simulink model "ev_pv_smoothing"  (Simulink 8.1)
settings: Solver=ode3  StartTime=0  StopTime=86400  FixedStep=15  RelTol=1e-3
undefined symbols (not defined in the file or in its folder): D1, Delta, SRRL, Ts, Weather
libraries: CampusEnergyModeling x22, powerlib x9, simulink x4, powerlib_meascontrol x4
settings Model: Creator=sfrank1  LastModifiedBy=sfrank1
settings DataIOCC: SignalLoggingSaveFormat=Dataset
settings OptimizationCC: ExpressionDepthLimit=128
settings DebuggingCC: FcnCallInpInsideContextMsg=EnableAllAsError
settings GRTTargetCC: CombineOutputUpdateFcns=on  GRTInterface=off

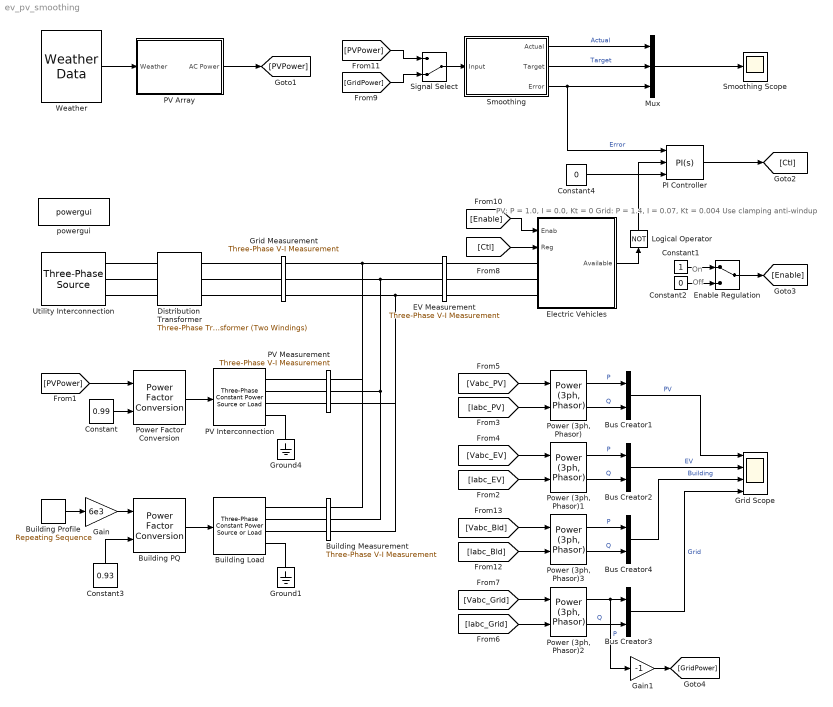
== system ev_pv_smoothing ==
  note: PV: P = 1.0, I = 0.0, Kt = 0
      | Grid: P = 1.4, I = 0.07, Kt = 0.004
      | Use clamping anti-windup
  note: Off
  note: On
  Building Measurement : powerlib/Measurements/Three-Phase V-I Measurement  VoltageMeasurement=phase-to-ground  SetLabelV=on  LabelV=Vabc_Bld  Vpu=off  VpuLL=off  CurrentMeasurement=yes  SetLabelI=on  LabelI=Iabc_Bld  Ipu=off  Pbase=100e3  Vbase=208e3  OutputType=Complex  PhasorSimulation=on  PSBequivalent=0
  Building Profile : simulink/Sources/Repeating Sequence  rep_seq_t=[0 1 2 3 4 5 6 7 8 9 10 11 12 13 14 15 16 17 18 19 20 21 22 23 24]*3600  rep_seq_y=[0.53 0.53 0.54 0.54 0.56 0.77 0.95 1.53 1.79 1.80 1.83 1.83 1.88 1.91 1.91 1.92 1.63 1.28 1.20 1.13 1.08 0.71 0.52 0.52 0.53]
  Building Load : CampusEnergyModeling/Electrical/Three-Phase Constant Power Source or Load  Conven=load  PNom=5e3  QNom=2e3  VNom=208  fNom=60  VLow=0.7
  Building PQ : CampusEnergyModeling/Electrical/Power Factor Conversion  pfType=Lagging
  Bus Creator{1..4} (4 alike) : BusCreator  Inputs=2
  Constant : Constant  Value=0.99
  Constant1 : Constant
  Constant2 : Constant  Value=0
  Constant3 : Constant  Value=0.93
  Constant4 : Constant  Value=0
  Distribution Transformer : powerlib/Elements/Three-Phase Transformer (Two Windings)  Winding1Connection=Delta (D1)  UNITS=pu  NominalPower=[10e3 , 60]  Winding1=[13.2e3 , 0.02/2 , 0.05/(120*pi)/2]  Winding2Connection=Yg  Winding2=[208, 0.02/2 , 0.05/(120*pi)/2]  SetSaturation=off  Rm=500  Lm=200  Saturation=[ 0,0 ; 0.0024,1.2 ; 1.0,1.52 ]  Hysteresis=off  DataFile='hysteresis'  SetInitialFlux=off  InitialFluxes=[ 0.8 , -0.8 , 0.7 ]  Measurements=None  MoreParameters=off  BreakLoop=off  DataType=off  TransfoNumber=1
  EV Measurement : powerlib/Measurements/Three-Phase V-I Measurement  VoltageMeasurement=phase-to-ground  SetLabelV=on  LabelV=Vabc_EV  Vpu=off  VpuLL=off  CurrentMeasurement=yes  SetLabelI=on  LabelI=Iabc_EV  Ipu=off  Pbase=100e3  Vbase=208e3  OutputType=Complex  PhasorSimulation=on  PSBequivalent=0
  Electric Vehicles : Subsystem
  Enable Regulation : ManualSwitch
  Gain : Gain  Gain=6e3
  Gain1 : Gain  Gain=-1
  Grid Measurement : powerlib/Measurements/Three-Phase V-I Measurement  VoltageMeasurement=phase-to-ground  SetLabelV=on  LabelV=Vabc_Grid  Vpu=off  VpuLL=off  CurrentMeasurement=yes  SetLabelI=on  LabelI=Iabc_Grid  Ipu=off  Pbase=100e3  Vbase=208e3  OutputType=Complex  PhasorSimulation=on  PSBequivalent=0
  Grid Scope : Scope  NumInputPorts=4
      settings: ShowLegends=on  TimeRange=86400  YMin=-5000~-5000~-5000~-5000  YMax=25000~25000~25000~25000
  Ground1 : powerlib/Elements/Ground  LConnTagsString=a
  Ground4 : powerlib/Elements/Ground  LConnTagsString=a
  Logical Operator : Logic  Operator=NOT  IconShape=distinctive  AllPortsSameDT=off  OutDataTypeStr=boolean
  Mux : Mux  Inputs=3
  PI Controller : simulink/Continuous/PID Controller  Controller=PI  TimeDomain=Continuous-time  SampleTime=1  IntegratorMethod=Forward Euler  FilterMethod=Forward Euler  Form=Parallel  P=1.4  I=0.07  D=0  N=100  InitialConditionSource=internal  InitialConditionForIntegrator=0  InitialConditionForFilter=0  ExternalReset=level  ZeroCross=off  LimitOutput=on  UpperSaturationLimit=12e3  LowerSaturationLimit=-12e3  LinearizeAsGain=on  AntiWindupMode=clamping  Kb=1  TrackingMode=on  Kt=0.004  PParamMin=[]  PParamMax=[]  IParamMin=[]  IParamMax=[]  DParamMin=[]  DParamMax=[]  NParamMin=[]  NParamMax=[]  KbParamMin=[]  KbParamMax=[]  KtParamMin=[]  KtParamMax=[]  POutMin=[]  POutMax=[]  IOutMin=[]  IOutMax=[]  DOutMin=[]  DOutMax=[]  NOutMin=[]  NOutMax=[]  KbOutMin=[]  KbOutMax=[]  KtOutMin=[]  KtOutMax=[]  IntegratorOutMin=[]  IntegratorOutMax=[]  FilterOutMin=[]  FilterOutMax=[]  SumOutMin=[]  SumOutMax=[]  SumI1OutMin=[]  SumI1OutMax=[]  SumI2OutMin=[]  SumI2OutMax=[]  SumI3OutMin=[]  SumI3OutMax=[]  SumDOutMin=[]  SumDOutMax=[]  SaturationOutMin=[]  SaturationOutMax=[]  IntegratorContinuousStateAttributes=''  IntegratorStateMustResolveToSignalObject=off  IntegratorRTWStateStorageClass=Auto  FilterContinuousStateAttributes=''  FilterStateMustResolveToSignalObject=off  FilterRTWStateStorageClass=Auto
  PV Interconnection : CampusEnergyModeling/Electrical/Three-Phase Constant Power Source or Load  Conven=source  PNom=20e3  QNom=0  VNom=208  fNom=60  VLow=0.7
  PV Array : Subsystem
  PV Measurement : powerlib/Measurements/Three-Phase V-I Measurement  VoltageMeasurement=phase-to-ground  SetLabelV=on  LabelV=Vabc_PV  Vpu=off  VpuLL=off  CurrentMeasurement=yes  SetLabelI=on  LabelI=Iabc_PV  Ipu=off  Pbase=100e3  Vbase=208e3  OutputType=Complex  PhasorSimulation=on  PSBequivalent=0
  Power (3ph, Phasor){,1..3} (4 alike) : powerlib_meascontrol/Measurements/Power (3ph, Phasor)
  Power Factor Conversion : CampusEnergyModeling/Electrical/Power Factor Conversion  pfType=Lagging
  Signal Select : ManualSwitch  CurrentSetting=0
  Smoothing : Subsystem
  Smoothing Scope : Scope
      settings: ShowLegends=on  TimeRange=86400  YMin=-20000  YMax=20000
  Utility Interconnection : powerlib/Electrical Sources/Three-Phase Source  Voltage=13.2e3  PhaseAngle=0  Frequency=60  InternalConnection=Yg  SpecifyImpedance=on  Resistance=0.8929  Inductance=16.58e-3  ShortCircuitLevel=1e6  BaseVoltage=13.2e3  XRratio=8  BusType=swing  Pref=0  Qref=0  Qmin=-inf  Qmax=inf
  Weather : CampusEnergyModeling/Weather/Weather Data  fname=Weather-SRRL.mat  initbus=on
  powergui : powerlib/powergui  Priority=2  SimulationMode=Phasor  SolverType=Tustin  SampleTime=Ts  frequency=60  SPID=off  DisableSnubberDevices=off  DisableRonSwitches=off  DisableVfSwitches=off  SwTol=0  Interpol=off  DisplayEquations=off  frequencyindice=60  Pbase=100e6  ErrMax=1e-4  Iterations=50  UnitsV=kV  UnitsW=kW  FunctionMessages=off  echomessages=off  HookPort=off  EnableUseOfTLC=off  x0status=blocks  RestoreLinks=warning  ResistiveCurrentMeasurement=off  Frange=[0:2:500]  Ylog=off  Xlog=on  ShowGrid=off  save=off  variable=ZData  structure=Sig1  ZoomFFT=on  StartTime=0.26  cycles=2  DisplayStyle=1  fundamental=60  FreqAxis=off  MaxFrequency=5000  frequencyindicesteady=1  RmsSteady=1  display=off  Ts=0  methode=off
  wires:
  Smoothing/3(Error) -> PI Controller/1, Mux/3  "Error"
  Mux/1 -> Smoothing Scope/1
  Smoothing/1(Actual) -> Mux/1  "Actual"
  Smoothing/2(Target) -> Mux/2  "Target"
  Constant/1 -> Power Factor Conversion/2
  Power Factor Conversion/1 -> PV Interconnection/1
  [Vabc_PV] -> "Power (3ph, Phasor)"/1
  [Iabc_PV] -> "Power (3ph, Phasor)"/2
  "Power (3ph, Phasor)"/2 -> Bus Creator1/2  "Q"
  "Power (3ph, Phasor)"/1 -> Bus Creator1/1  "P"
  Bus Creator1/1 -> Grid Scope/1  "PV"
  [Vabc_EV] -> "Power (3ph, Phasor)1"/1
  [Iabc_EV] -> "Power (3ph, Phasor)1"/2
  "Power (3ph, Phasor)1"/2 -> Bus Creator2/2  "Q"
  "Power (3ph, Phasor)1"/1 -> Bus Creator2/1  "P"
  [Vabc_Grid] -> "Power (3ph, Phasor)2"/1
  [Iabc_Grid] -> "Power (3ph, Phasor)2"/2
  "Power (3ph, Phasor)2"/2 -> Bus Creator3/2  "Q"
  "Power (3ph, Phasor)2"/1 -> Gain1/1, Bus Creator3/1  "P"
  Bus Creator3/1 -> Grid Scope/4  "Grid"
  Bus Creator2/1 -> Grid Scope/2  "EV"
  Constant1/1 -> Enable Regulation/1
  Constant2/1 -> Enable Regulation/2
  Weather/1 -> PV Array/1(Weather)
  [PVPower] -> Power Factor Conversion/1
  [Ctl] -> Electric Vehicles/2(Reg)
  Enable Regulation/1 -> [Enable]
  [Enable] -> Electric Vehicles/1(Enab)
  Building PQ/1 -> Building Load/1
  Building Profile/1 -> Gain/1
  [Vabc_Bld] -> "Power (3ph, Phasor)3"/1
  [Iabc_Bld] -> "Power (3ph, Phasor)3"/2
  "Power (3ph, Phasor)3"/2 -> Bus Creator4/2  "Q"
  "Power (3ph, Phasor)3"/1 -> Bus Creator4/1  "P"
  Bus Creator4/1 -> Grid Scope/3  "Building"
  Gain/1 -> Building PQ/1
  Constant3/1 -> Building PQ/2
  Electric Vehicles/1(Available) -> Logical Operator/1
  Signal Select/1 -> Smoothing/1(Input)
  [PVPower] -> Signal Select/1
  [GridPower] -> Signal Select/2
  Logical Operator/1 -> PI Controller/2
  PI Controller/1 -> [Ctl]
  Gain1/1 -> [GridPower]
  PV Array/1(AC Power) -> [PVPower]
  Constant4/1 -> PI Controller/3
  connections:
  Utility Interconnection/RConn1 -- Distribution Transformer/LConn1
  Distribution Transformer/LConn2 -- Utility Interconnection/RConn2
  Utility Interconnection/RConn3 -- Distribution Transformer/LConn3
  EV Measurement/LConn1 -- Building Measurement/LConn1 -- PV Measurement/RConn1 -- Grid Measurement/RConn1
  PV Measurement/RConn2 -- EV Measurement/LConn2 -- Grid Measurement/RConn2 -- Building Measurement/LConn2
  EV Measurement/LConn3 -- Building Measurement/LConn3 -- PV Measurement/RConn3 -- Grid Measurement/RConn3
  PV Interconnection/RConn4 -- Ground4/LConn1
  PV Measurement/LConn1 -- PV Interconnection/RConn1
  PV Measurement/LConn2 -- PV Interconnection/RConn2
  PV Measurement/LConn3 -- PV Interconnection/RConn3
  EV Measurement/RConn1 -- Electric Vehicles/LConn1
  EV Measurement/RConn2 -- Electric Vehicles/LConn2
  EV Measurement/RConn3 -- Electric Vehicles/LConn3
  Building Load/RConn4 -- Ground1/LConn1
  Distribution Transformer/RConn1 -- Grid Measurement/LConn1
  Distribution Transformer/RConn2 -- Grid Measurement/LConn2
  Distribution Transformer/RConn3 -- Grid Measurement/LConn3
  Building Load/RConn1 -- Building Measurement/RConn1
  Building Load/RConn2 -- Building Measurement/RConn2
  Building Load/RConn3 -- Building Measurement/RConn3

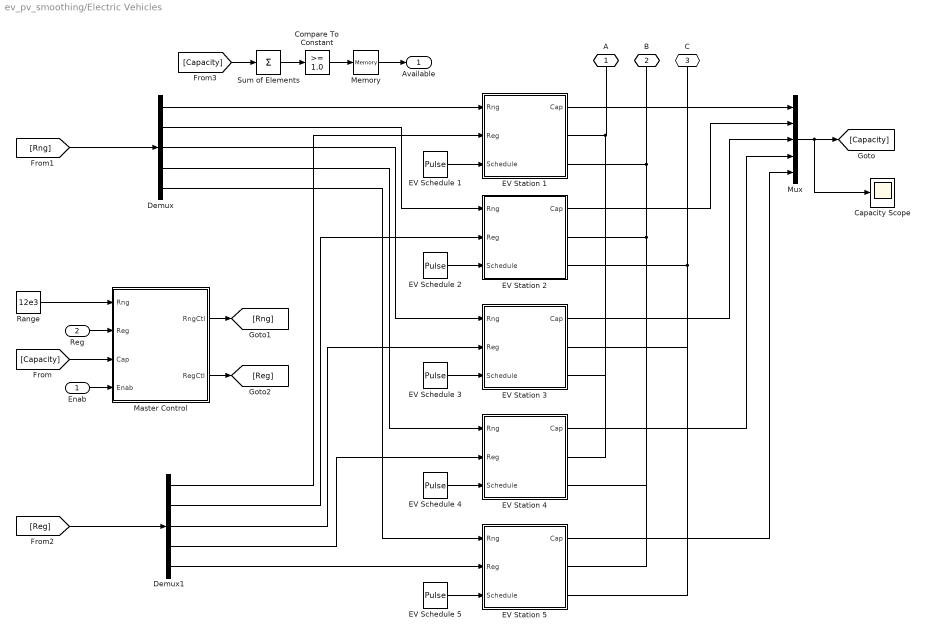
== system ev_pv_smoothing/Electric Vehicles ==
  Enab : Inport
  Reg : Inport  Port=2
  Capacity Scope : Scope
      settings: ShowLegends=on  TimeRange=86400  YMin=0  YMax=3000  SaveName=ScopeData3
  Compare To Constant : simulink/Logic and Bit Operations/Compare To Constant  relop=>=  const=1.0  OutDataTypeStr=boolean
  Demux : Demux  Outputs=5
  Demux1 : Demux  Outputs=5
  EV Schedule 1 : DiscretePulseGenerator  PulseType=Time based  Period=86400  PulseWidth=(9/24)*100  PhaseDelay=(6)*3600
  EV Schedule 2 : DiscretePulseGenerator  PulseType=Time based  Period=86400  PulseWidth=(9/24)*100  PhaseDelay=(6.5)*3600
  EV Schedule 3 : DiscretePulseGenerator  PulseType=Time based  Period=86400  PulseWidth=(9/24)*100  PhaseDelay=(7)*3600
  EV Schedule 4 : DiscretePulseGenerator  PulseType=Time based  Period=86400  PulseWidth=(9/24)*100  PhaseDelay=(7.5)*3600
  EV Schedule 5 : DiscretePulseGenerator  PulseType=Time based  Period=86400  PulseWidth=(9/24)*100  PhaseDelay=(8)*3600
  EV Station 1 : Subsystem
  EV Station 2 : Subsystem
  EV Station 3 : Subsystem
  EV Station 4 : Subsystem
  EV Station 5 : Subsystem
  Master Control : Subsystem
  Memory : Memory
  Mux : Mux  Inputs=5
  Range : Constant  Value=12e3
  Sum of Elements : Sum  Inputs=+
  A : PMIOPort  Port=1  Side=Left
  B : PMIOPort  Port=2  Side=Left
  C : PMIOPort  Port=3  Side=Left
  Available : Outport
  wires:
  EV Schedule 1/1 -> EV Station 1/3(Schedule)
  EV Schedule 2/1 -> EV Station 2/3(Schedule)
  EV Schedule 3/1 -> EV Station 3/3(Schedule)
  EV Schedule 4/1 -> EV Station 4/3(Schedule)
  EV Schedule 5/1 -> EV Station 5/3(Schedule)
  Range/1 -> Master Control/1(Rng)
  Reg/1 -> Master Control/2(Reg)
  Enab/1 -> Master Control/4(Enab)
  EV Station 1/1(Cap) -> Mux/1
  EV Station 2/1(Cap) -> Mux/2
  EV Station 3/1(Cap) -> Mux/3
  EV Station 4/1(Cap) -> Mux/4
  EV Station 5/1(Cap) -> Mux/5
  Mux/1 -> Capacity Scope/1, [Capacity]
  [Capacity] -> Master Control/3(Cap)
  Master Control/2(RegCtl) -> [Reg]
  Master Control/1(RngCtl) -> [Rng]
  [Rng] -> Demux/1
  [Reg] -> Demux1/1
  Demux/1 -> EV Station 1/1(Rng)
  Demux1/5 -> EV Station 5/2(Reg)
  Demux/2 -> EV Station 2/1(Rng)
  Demux/3 -> EV Station 3/1(Rng)
  Demux/4 -> EV Station 4/1(Rng)
  Demux/5 -> EV Station 5/1(Rng)
  Demux1/1 -> EV Station 1/2(Reg)
  Demux1/2 -> EV Station 2/2(Reg)
  Demux1/3 -> EV Station 3/2(Reg)
  Demux1/4 -> EV Station 4/2(Reg)
  Sum of Elements/1 -> Compare To Constant/1
  [Capacity] -> Sum of Elements/1
  Compare To Constant/1 -> Memory/1
  Memory/1 -> Available/1
  connections:
  EV Station 1/RConn2 -- EV Station 2/RConn1 -- EV Station 5/RConn1 -- EV Station 4/RConn2 -- B/RConn1
  EV Station 5/RConn2 -- EV Station 3/RConn1 -- EV Station 2/RConn2 -- C/RConn1
  EV Station 1/RConn1 -- EV Station 4/RConn1 -- EV Station 3/RConn2 -- A/RConn1

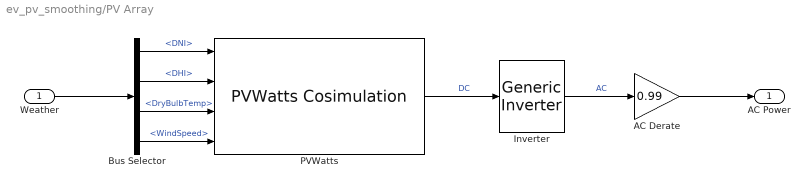
== system ev_pv_smoothing/PV Array ==
  Weather : Inport
  AC Derate : Gain  Gain=0.99
  Bus Selector : BusSelector  OutputSignals=DNI,DHI,DryBulbTemp,WindSpeed
  Inverter : CampusEnergyModeling/PV/Generic Inverter  max_power=20.0e3  standby=10.0  model_type=Fixed Efficiency  fixed_eff=0.96  alpha=100.0  beta=0.04  gamma=4.0e-07  lookup_pair=Input Power + Output Power  lookup_in=[0, 10, 25, 50, 75, 100]  lookup_out=[0, 9, 24, 49, 73, 97]  lookup_eff=[0.10, 0.80, 0.87, 0.93, 0.90, 0.88]
  PVWatts : CampusEnergyModeling/PV/PVWatts Cosimulation  lat=39.7  lon=-105.2  start_time=2012-05-17 00:00:00  tz=-7  time_step=15  system_size=20.0e3  derate=0.908  azimuth=180  tilt=10  use_lat_tilt=off  track_mode=Fixed  rotlim=45  use_cell_data=off  t_ref=25  t_noct=45  gamma=-0.5  i_ref=1000  poa_cutin=0  init_tcell=16.8  init_poa=0  alignment=Middle  output_dc=on  output_celltemp=off  output_poa=off
  AC Power : Outport
  wires:
  Bus Selector/1 -> PVWatts/1  "<DNI>"
  Bus Selector/2 -> PVWatts/2  "<DHI>"
  Bus Selector/3 -> PVWatts/3  "<DryBulbTemp>"
  Bus Selector/4 -> PVWatts/4  "<WindSpeed>"
  PVWatts/1 -> Inverter/1  "DC"
  Inverter/1 -> AC Derate/1  "AC"
  AC Derate/1 -> AC Power/1
  Weather/1 -> Bus Selector/1

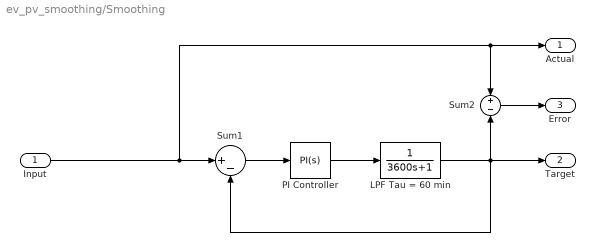
== system ev_pv_smoothing/Smoothing ==
  Input : Inport
  LPF Tau = 60 min : TransferFcn  Denominator=[3600 1]
  PI Controller : simulink/Continuous/PID Controller  Controller=PI  TimeDomain=Continuous-time  SampleTime=1  IntegratorMethod=Forward Euler  FilterMethod=Forward Euler  Form=Parallel  P=0.80  I=0.001  D=0  N=100  InitialConditionSource=internal  InitialConditionForIntegrator=0  InitialConditionForFilter=0  ExternalReset=none  LimitOutput=off  UpperSaturationLimit=20e3  LowerSaturationLimit=-20e3  LinearizeAsGain=on  AntiWindupMode=back-calculation  Kb=1  TrackingMode=off  Kt=1  PParamMin=[]  PParamMax=[]  IParamMin=[]  IParamMax=[]  DParamMin=[]  DParamMax=[]  NParamMin=[]  NParamMax=[]  KbParamMin=[]  KbParamMax=[]  KtParamMin=[]  KtParamMax=[]  POutMin=[]  POutMax=[]  IOutMin=[]  IOutMax=[]  DOutMin=[]  DOutMax=[]  NOutMin=[]  NOutMax=[]  KbOutMin=[]  KbOutMax=[]  KtOutMin=[]  KtOutMax=[]  IntegratorOutMin=[]  IntegratorOutMax=[]  FilterOutMin=[]  FilterOutMax=[]  SumOutMin=[]  SumOutMax=[]  SumI1OutMin=[]  SumI1OutMax=[]  SumI2OutMin=[]  SumI2OutMax=[]  SumI3OutMin=[]  SumI3OutMax=[]  SumDOutMin=[]  SumDOutMax=[]  SaturationOutMin=[]  SaturationOutMax=[]  IntegratorContinuousStateAttributes=''  IntegratorStateMustResolveToSignalObject=off  IntegratorRTWStateStorageClass=Auto  FilterContinuousStateAttributes=''  FilterStateMustResolveToSignalObject=off  FilterRTWStateStorageClass=Auto
  Sum1 : Sum  Inputs=|+-
  Sum2 : Sum  Inputs=+-
  Actual : Outport
  Target : Outport  Port=2
  Error : Outport  Port=3
  wires:
  Sum2/1 -> Error/1
  LPF Tau = 60 min/1 -> Sum1/2, Target/1, Sum2/2
  Input/1 -> Sum2/1, Actual/1, Sum1/1
  PI Controller/1 -> LPF Tau = 60 min/1
  Sum1/1 -> PI Controller/1

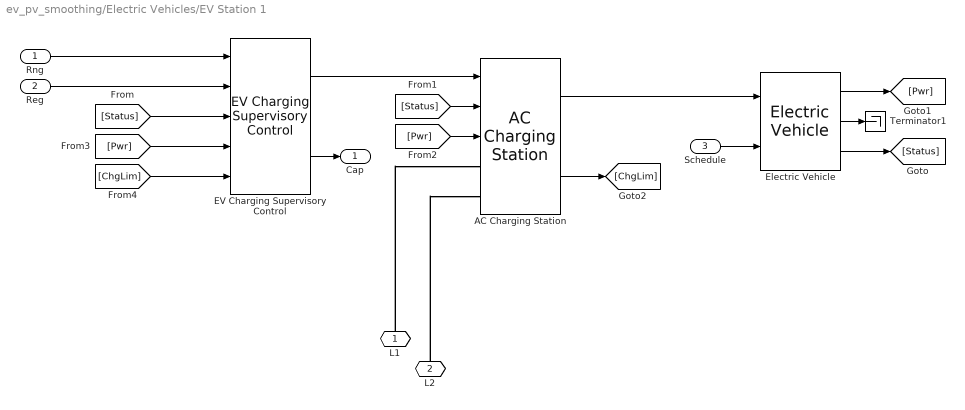
== system ev_pv_smoothing/Electric Vehicles/EV Station 1 ==
  Rng : Inport
  Reg : Inport  Port=2
  Schedule : Inport  Port=3
  AC Charging Station : CampusEnergyModeling/Electric Vehicles/AC Charging Station  prated=6600  vrated=240  pstandby=50  eff=0.99  pf=0.99  freq=60
  EV Charging Supervisory Control : CampusEnergyModeling/Electric Vehicles/EV Charging Supervisory Control  ctype=AC  ramp=100  regtype=Two-sided  ldsettings=on  sweepint=1650+300*rand(1)  sweepramp=10  thr=1.0
  Electric Vehicle : CampusEnergyModeling/Electric Vehicles/Electric Vehicle  ctype=AC  rating=6240  chargerEff=0.96  profile=off  profileSOC=[0.00 0.10 0.20 0.80 0.99 1.00]  profileRate=[0.10 0.20 1.00 1.00 0.01 0.00]  capacity=24000  initSOC=0.3  battEff=0.98
  Terminator1 : Terminator
  L1 : PMIOPort  Port=1  Side=Right
  L2 : PMIOPort  Port=2  Side=Right
  Cap : Outport
  wires:
  AC Charging Station/1 -> Electric Vehicle/1
  Schedule/1 -> Electric Vehicle/2
  Electric Vehicle/3 -> [Status]
  [Status] -> EV Charging Supervisory Control/3
  Electric Vehicle/1 -> [Pwr]
  EV Charging Supervisory Control/1 -> AC Charging Station/1
  [Status] -> AC Charging Station/2
  [Pwr] -> AC Charging Station/3
  Reg/1 -> EV Charging Supervisory Control/2
  Rng/1 -> EV Charging Supervisory Control/1
  EV Charging Supervisory Control/2 -> Cap/1
  Electric Vehicle/2 -> Terminator1/1
  [Pwr] -> EV Charging Supervisory Control/4
  [ChgLim] -> EV Charging Supervisory Control/5
  AC Charging Station/2 -> [ChgLim]
  connections:
  L1/RConn1 -- AC Charging Station/LConn1
  L2/RConn1 -- AC Charging Station/LConn2

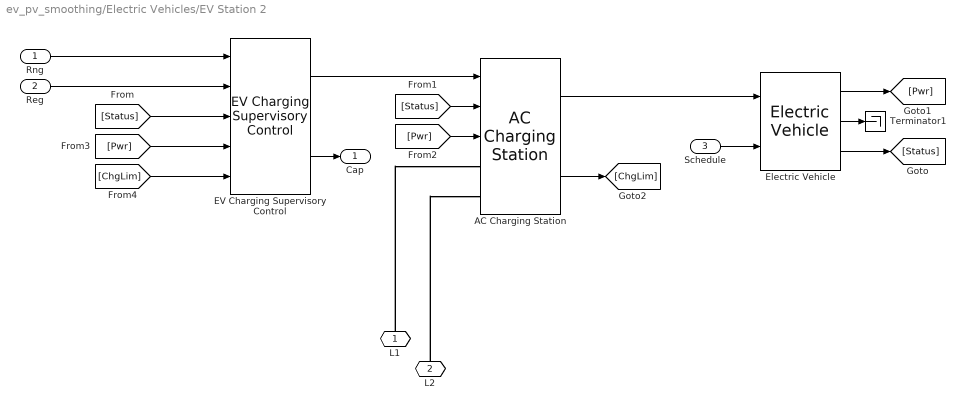
== system ev_pv_smoothing/Electric Vehicles/EV Station 2 ==
  Rng : Inport
  Reg : Inport  Port=2
  Schedule : Inport  Port=3
  AC Charging Station : CampusEnergyModeling/Electric Vehicles/AC Charging Station  prated=6600  vrated=240  pstandby=50  eff=0.99  pf=0.99  freq=60
  EV Charging Supervisory Control : CampusEnergyModeling/Electric Vehicles/EV Charging Supervisory Control  ctype=AC  ramp=100  regtype=Two-sided  ldsettings=on  sweepint=1650+300*rand(1)  sweepramp=10  thr=1.0
  Electric Vehicle : CampusEnergyModeling/Electric Vehicles/Electric Vehicle  ctype=AC  rating=6240  chargerEff=0.96  profile=off  profileSOC=[0.00 0.10 0.20 0.80 0.99 1.00]  profileRate=[0.10 0.20 1.00 1.00 0.01 0.00]  capacity=24000  initSOC=0.3  battEff=0.98
  Terminator1 : Terminator
  L1 : PMIOPort  Port=1  Side=Right
  L2 : PMIOPort  Port=2  Side=Right
  Cap : Outport
  wires:
  AC Charging Station/1 -> Electric Vehicle/1
  Schedule/1 -> Electric Vehicle/2
  Electric Vehicle/3 -> [Status]
  [Status] -> EV Charging Supervisory Control/3
  Electric Vehicle/1 -> [Pwr]
  EV Charging Supervisory Control/1 -> AC Charging Station/1
  [Status] -> AC Charging Station/2
  [Pwr] -> AC Charging Station/3
  Reg/1 -> EV Charging Supervisory Control/2
  Rng/1 -> EV Charging Supervisory Control/1
  EV Charging Supervisory Control/2 -> Cap/1
  Electric Vehicle/2 -> Terminator1/1
  [Pwr] -> EV Charging Supervisory Control/4
  [ChgLim] -> EV Charging Supervisory Control/5
  AC Charging Station/2 -> [ChgLim]
  connections:
  L1/RConn1 -- AC Charging Station/LConn1
  L2/RConn1 -- AC Charging Station/LConn2

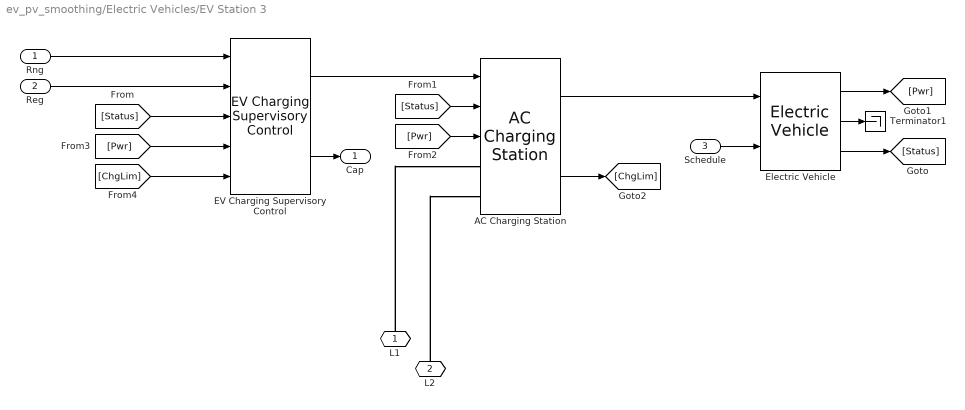
== system ev_pv_smoothing/Electric Vehicles/EV Station 3 ==
  Rng : Inport
  Reg : Inport  Port=2
  Schedule : Inport  Port=3
  AC Charging Station : CampusEnergyModeling/Electric Vehicles/AC Charging Station  prated=6600  vrated=240  pstandby=50  eff=0.99  pf=0.99  freq=60
  EV Charging Supervisory Control : CampusEnergyModeling/Electric Vehicles/EV Charging Supervisory Control  ctype=AC  ramp=100  regtype=Two-sided  ldsettings=on  sweepint=1650+300*rand(1)  sweepramp=10  thr=1.0
  Electric Vehicle : CampusEnergyModeling/Electric Vehicles/Electric Vehicle  ctype=AC  rating=6240  chargerEff=0.96  profile=off  profileSOC=[0.00 0.10 0.20 0.80 0.99 1.00]  profileRate=[0.10 0.20 1.00 1.00 0.01 0.00]  capacity=24000  initSOC=0.3  battEff=0.98
  Terminator1 : Terminator
  L1 : PMIOPort  Port=1  Side=Right
  L2 : PMIOPort  Port=2  Side=Right
  Cap : Outport
  wires:
  AC Charging Station/1 -> Electric Vehicle/1
  Schedule/1 -> Electric Vehicle/2
  Electric Vehicle/3 -> [Status]
  [Status] -> EV Charging Supervisory Control/3
  Electric Vehicle/1 -> [Pwr]
  EV Charging Supervisory Control/1 -> AC Charging Station/1
  [Status] -> AC Charging Station/2
  [Pwr] -> AC Charging Station/3
  Reg/1 -> EV Charging Supervisory Control/2
  Rng/1 -> EV Charging Supervisory Control/1
  EV Charging Supervisory Control/2 -> Cap/1
  Electric Vehicle/2 -> Terminator1/1
  [Pwr] -> EV Charging Supervisory Control/4
  [ChgLim] -> EV Charging Supervisory Control/5
  AC Charging Station/2 -> [ChgLim]
  connections:
  L1/RConn1 -- AC Charging Station/LConn1
  L2/RConn1 -- AC Charging Station/LConn2

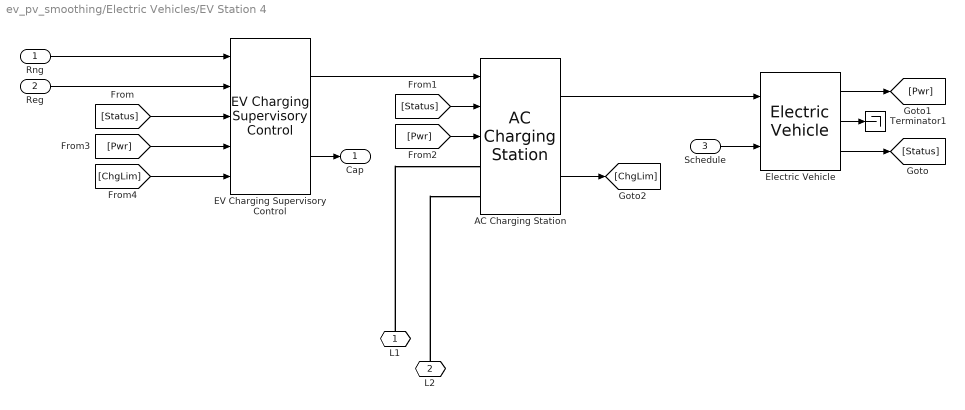
== system ev_pv_smoothing/Electric Vehicles/EV Station 4 ==
  Rng : Inport
  Reg : Inport  Port=2
  Schedule : Inport  Port=3
  AC Charging Station : CampusEnergyModeling/Electric Vehicles/AC Charging Station  prated=6600  vrated=240  pstandby=50  eff=0.99  pf=0.99  freq=60
  EV Charging Supervisory Control : CampusEnergyModeling/Electric Vehicles/EV Charging Supervisory Control  ctype=AC  ramp=100  regtype=Two-sided  ldsettings=on  sweepint=1650+300*rand(1)  sweepramp=10  thr=1.0
  Electric Vehicle : CampusEnergyModeling/Electric Vehicles/Electric Vehicle  ctype=AC  rating=6240  chargerEff=0.96  profile=off  profileSOC=[0.00 0.10 0.20 0.80 0.99 1.00]  profileRate=[0.10 0.20 1.00 1.00 0.01 0.00]  capacity=24000  initSOC=0.3  battEff=0.98
  Terminator1 : Terminator
  L1 : PMIOPort  Port=1  Side=Right
  L2 : PMIOPort  Port=2  Side=Right
  Cap : Outport
  wires:
  AC Charging Station/2 -> [ChgLim]
  [ChgLim] -> EV Charging Supervisory Control/5
  [Pwr] -> EV Charging Supervisory Control/4
  Electric Vehicle/2 -> Terminator1/1
  EV Charging Supervisory Control/2 -> Cap/1
  Rng/1 -> EV Charging Supervisory Control/1
  Reg/1 -> EV Charging Supervisory Control/2
  [Pwr] -> AC Charging Station/3
  [Status] -> AC Charging Station/2
  EV Charging Supervisory Control/1 -> AC Charging Station/1
  Electric Vehicle/1 -> [Pwr]
  [Status] -> EV Charging Supervisory Control/3
  Electric Vehicle/3 -> [Status]
  Schedule/1 -> Electric Vehicle/2
  AC Charging Station/1 -> Electric Vehicle/1
  connections:
  L2/RConn1 -- AC Charging Station/LConn2
  L1/RConn1 -- AC Charging Station/LConn1

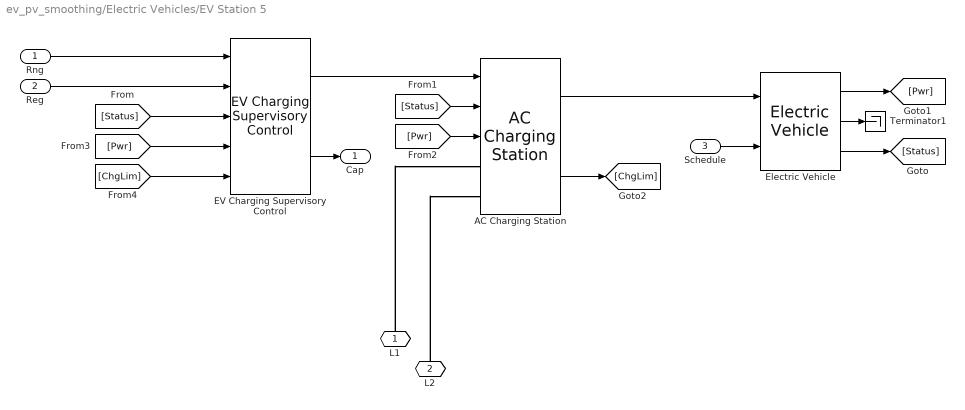
== system ev_pv_smoothing/Electric Vehicles/EV Station 5 ==
  Rng : Inport
  Reg : Inport  Port=2
  Schedule : Inport  Port=3
  AC Charging Station : CampusEnergyModeling/Electric Vehicles/AC Charging Station  prated=6600  vrated=240  pstandby=50  eff=0.99  pf=0.99  freq=60
  EV Charging Supervisory Control : CampusEnergyModeling/Electric Vehicles/EV Charging Supervisory Control  ctype=AC  ramp=100  regtype=Two-sided  ldsettings=on  sweepint=1650+300*rand(1)  sweepramp=10  thr=1.0
  Electric Vehicle : CampusEnergyModeling/Electric Vehicles/Electric Vehicle  ctype=AC  rating=6240  chargerEff=0.96  profile=off  profileSOC=[0.00 0.10 0.20 0.80 0.99 1.00]  profileRate=[0.10 0.20 1.00 1.00 0.01 0.00]  capacity=24000  initSOC=0.3  battEff=0.98
  Terminator1 : Terminator
  L1 : PMIOPort  Port=1  Side=Right
  L2 : PMIOPort  Port=2  Side=Right
  Cap : Outport
  wires:
  AC Charging Station/1 -> Electric Vehicle/1
  Schedule/1 -> Electric Vehicle/2
  Electric Vehicle/3 -> [Status]
  [Status] -> EV Charging Supervisory Control/3
  Electric Vehicle/1 -> [Pwr]
  EV Charging Supervisory Control/1 -> AC Charging Station/1
  [Status] -> AC Charging Station/2
  [Pwr] -> AC Charging Station/3
  Reg/1 -> EV Charging Supervisory Control/2
  Rng/1 -> EV Charging Supervisory Control/1
  EV Charging Supervisory Control/2 -> Cap/1
  Electric Vehicle/2 -> Terminator1/1
  [Pwr] -> EV Charging Supervisory Control/4
  [ChgLim] -> EV Charging Supervisory Control/5
  AC Charging Station/2 -> [ChgLim]
  connections:
  L1/RConn1 -- AC Charging Station/LConn1
  L2/RConn1 -- AC Charging Station/LConn2

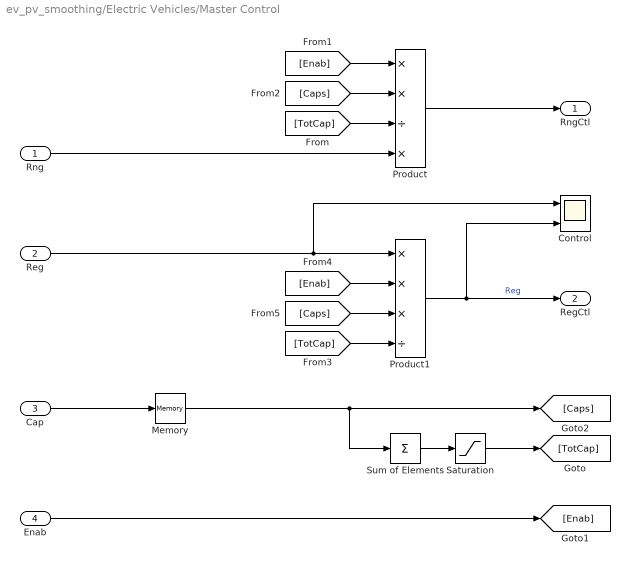
== system ev_pv_smoothing/Electric Vehicles/Master Control ==
  Rng : Inport
  Reg : Inport  Port=2
  Cap : Inport  Port=3
  Enab : Inport  Port=4
  Control : Scope  NumInputPorts=2
      settings: ShowLegends=on  TimeRange=86400  YMin=-15000~-10000  YMax=15000~15000  SaveName=ScopeData2
  Memory : Memory
  Product : Product  Inputs=**/*
  Product1 : Product  Inputs=***/
  Saturation : Saturate  UpperLimit=inf  LowerLimit=1
  Sum of Elements : Sum  Inputs=+
  RngCtl : Outport
  RegCtl : Outport  Port=2
  wires:
  Sum of Elements/1 -> Saturation/1
  Enab/1 -> [Enab]
  [TotCap] -> Product/3
  Rng/1 -> Product/4
  [TotCap] -> Product1/4
  [Enab] -> Product1/2
  [Caps] -> Product1/3
  [Enab] -> Product/1
  [Caps] -> Product/2
  Saturation/1 -> [TotCap]
  Product/1 -> RngCtl/1
  Product1/1 -> Control/2, RegCtl/1  "Reg"
  Reg/1 -> Control/1, Product1/1
  Memory/1 -> Sum of Elements/1, [Caps]
  Cap/1 -> Memory/1
